simulink model "exo5"  (R2020b)
settings: Solver=VariableStepAuto  StartTime=0.0  StopTime=204.5  RelTol=1e-3
values from neighbouring files (symbols this model uses):
  Te = 0.1    [exo5_mfile - Copy.m]    (also in exo5_mfile.m)
settings Model: Creator=alex  LastModifiedBy=alex

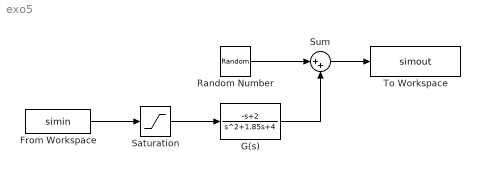
== system exo5 ==
  From Workspace : FromWorkspace  VariableName=simin  SampleTime=Te
  G(s) : TransferFcn  Numerator=[-1 2]  Denominator=[1 1.85 4]
  Random Number : RandomNumber  Variance=0.01  SampleTime=Te
  Saturation : Saturate
  Sum : Sum  Inputs=|++
  To Workspace : ToWorkspace  VariableName=simout  SaveFormat=Timeseries  SampleTime=Te
  wires:
  Saturation/1 -> G(s)/1
  Random Number/1 -> Sum/1
  G(s)/1 -> Sum/2
  From Workspace/1 -> Saturation/1
  Sum/1 -> To Workspace/1
